simulink model "ryll"  (R2015b)
settings: Solver=FixedStepAuto  StartTime=0  StopTime=8.9  FixedStep=10*(1e-4)  RelTol=1e-3
undefined symbols (not defined in the file or in its folder): qc
libraries: simulink x2
settings Model: Creator=acsl  LastModifiedBy=acsl

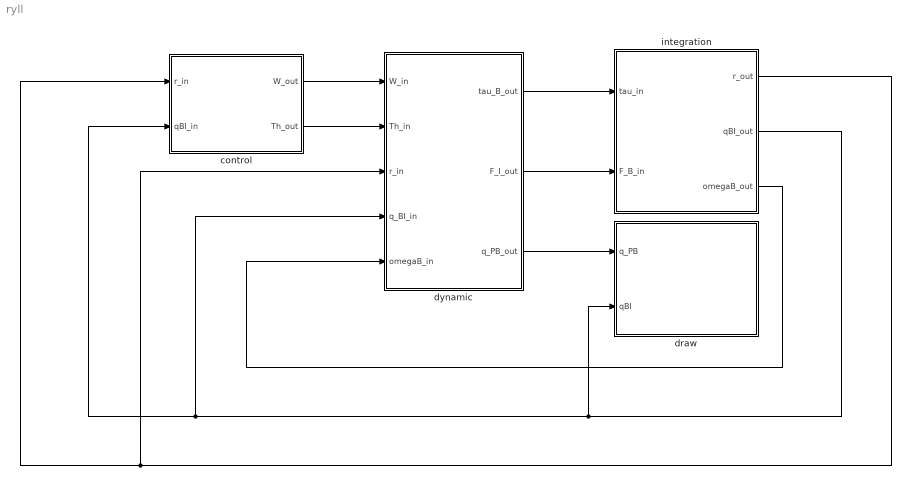
== system ryll ==
  control : Subsystem  InitFcn=init
  draw : Subsystem
  dynamic : Subsystem  StopFcn=close all
  integration : Subsystem
  wires:
  integration/1(r_out) -> dynamic/3(r_in), control/1(r_in)
  control/1(W_out) -> dynamic/1(W_in)
  control/2(Th_out) -> dynamic/2(Th_in)
  dynamic/2(F_I_out) -> integration/2(F_B_in)
  dynamic/1(tau_B_out) -> integration/1(tau_in)
  integration/3(omegaB_out) -> dynamic/5(omegaB_in)
  integration/2(qBI_out) -> draw/2(qBI), dynamic/4(q_BI_in), control/2(qBI_in)
  dynamic/3(q_PB_out) -> draw/1(q_PB)

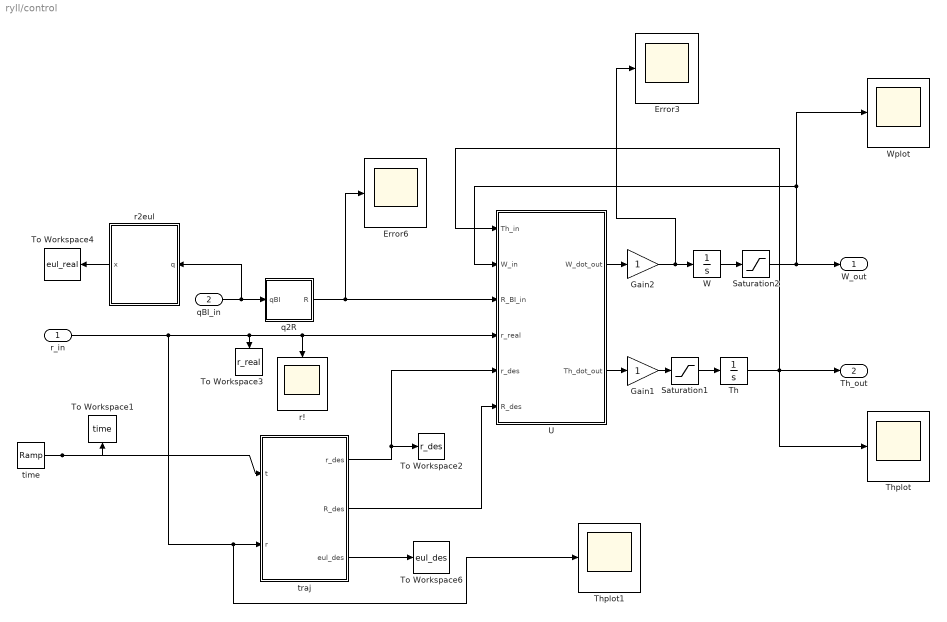
== system ryll/control ==
  r_in : Inport
  qBI_in : Inport  Port=2
  Error3 : Scope
  Error6 : Scope
  Gain1 : Gain
  Gain2 : Gain
  Saturation1 : Saturate  UpperLimit=qc.Th_dot_lim  LowerLimit=-qc.Th_dot_lim
  Saturation2 : Saturate  UpperLimit=qc.W_lim  LowerLimit=-qc.W_lim
  Th : Integrator  InitialCondition=qc.Th0
  Thplot : Scope
  Thplot1 : Scope
  To Workspace1 : ToWorkspace  VariableName=time  SaveFormat=Timeseries  SampleTime=-1
  To Workspace2 : ToWorkspace  VariableName=r_des  SaveFormat=Timeseries  SampleTime=-1
  To Workspace3 : ToWorkspace  VariableName=r_real  SaveFormat=Timeseries  SampleTime=-1
  To Workspace4 : ToWorkspace  VariableName=eul_real  SaveFormat=Timeseries  SampleTime=-1
  To Workspace6 : ToWorkspace  VariableName=eul_des  SaveFormat=Timeseries  SampleTime=-1
  U : Subsystem
  W : Integrator  InitialCondition=qc.W0
  Wplot : Scope
  q2R : MATLAB Function  TreatAsAtomicUnit=on
  r! : Scope
  r2eul : MATLAB Function  TreatAsAtomicUnit=on
  time : simulink/Sources/Ramp  slope=1  start=0  X0=0
  traj : MATLAB Function  TreatAsAtomicUnit=on
  W_out : Outport
  Th_out : Outport  Port=2
  wires:
  U/2(Th_dot_out) -> Gain1/1
  U/1(W_dot_out) -> Gain2/1
  W/1 -> Saturation2/1
  Gain1/1 -> Saturation1/1
  Th/1 -> U/1(Th_in), Th_out/1, Thplot/1
  Saturation1/1 -> Th/1
  Gain2/1 -> Error3/1, W/1
  time/1 -> traj/1(t), To Workspace1/1
  traj/2(R_des) -> U/6(R_des)
  q2R/1(R) -> Error6/1, U/3(R_BI_in)
  r_in/1 -> Thplot1/1, traj/2(r), r!/1, U/4(r_real), To Workspace3/1
  r2eul/1(x) -> To Workspace4/1
  traj/3(eul_des) -> To Workspace6/1
  qBI_in/1 -> r2eul/1(q), q2R/1(qBI)
  traj/1(r_des) -> U/5(r_des), To Workspace2/1
  Saturation2/1 -> U/2(W_in), Wplot/1, W_out/1

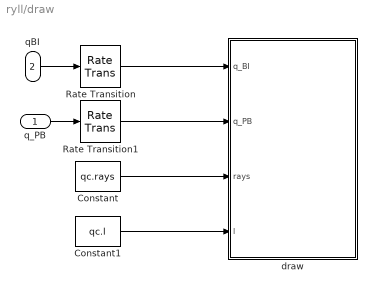
== system ryll/draw ==
  q_PB : Inport
  qBI : Inport  Port=2
  Constant : Constant  Value=qc.rays
  Constant1 : Constant  Value=qc.l
  Rate Transition : RateTransition
  Rate Transition1 : RateTransition
  draw : MATLAB Function  TreatAsAtomicUnit=on  SystemSampleTime=qc.draw_tick
  wires:
  Constant1/1 -> draw/4(l)
  q_PB/1 -> Rate Transition1/1
  Rate Transition1/1 -> draw/2(q_PB)
  Constant/1 -> draw/3(rays)
  Rate Transition/1 -> draw/1(q_BI)
  qBI/1 -> Rate Transition/1

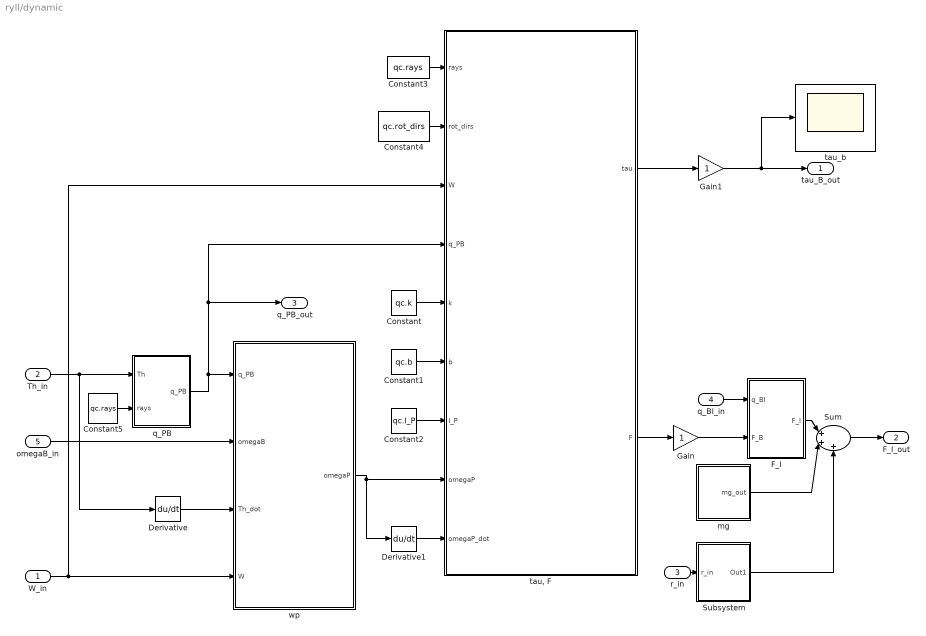
== system ryll/dynamic ==
  W_in : Inport
  Th_in : Inport  Port=2
  r_in : Inport  Port=3
  q_BI_in : Inport  Port=4
  omegaB_in : Inport  Port=5
  Constant : Constant  Value=qc.k
  Constant1 : Constant  Value=qc.b
  Constant2 : Constant  Value=qc.I_P
  Constant3 : Constant  Value=qc.rays
  Constant4 : Constant  Value=qc.rot_dirs
  Constant5 : Constant  Value=qc.rays
  Derivative : Derivative
  Derivative1 : Derivative
  F_I : MATLAB Function  TreatAsAtomicUnit=on
  Gain : Gain
  Gain1 : Gain
  Subsystem : Subsystem
  Sum : Sum  Inputs=|+++
  mg : Subsystem
  q_PB : MATLAB Function  TreatAsAtomicUnit=on
  "tau, F" : MATLAB Function  TreatAsAtomicUnit=on
  tau_b : Scope
  wp : MATLAB Function  TreatAsAtomicUnit=on
  tau_B_out : Outport
  F_I_out : Outport  Port=2
  q_PB_out : Outport  Port=3
  wires:
  Th_in/1 -> q_PB/1(Th), Derivative/1
  q_PB/1(q_PB) -> "tau, F"/4(q_PB), q_PB_out/1, wp/1(q_PB)
  omegaB_in/1 -> wp/2(omegaB)
  Derivative/1 -> wp/3(Th_dot)
  W_in/1 -> "tau, F"/3(W), wp/4(W)
  wp/1(omegaP) -> Derivative1/1, "tau, F"/8(omegaP)
  Constant/1 -> "tau, F"/5(k)
  Constant1/1 -> "tau, F"/6(b)
  Constant2/1 -> "tau, F"/7(I_P)
  "tau, F"/2(F) -> Gain/1
  Constant3/1 -> "tau, F"/1(rays)
  Constant4/1 -> "tau, F"/2(rot_dirs)
  Gain1/1 -> tau_b/1, tau_B_out/1
  Constant5/1 -> q_PB/2(rays)
  q_BI_in/1 -> F_I/1(q_BI)
  Gain/1 -> F_I/2(F_B)
  F_I/1(F_I) -> Sum/1
  mg/1(mg_out) -> Sum/2
  Sum/1 -> F_I_out/1
  r_in/1 -> Subsystem/1(r_in)
  Subsystem/1(Out1) -> Sum/3
  "tau, F"/1(tau) -> Gain1/1
  Derivative1/1 -> "tau, F"/9(omegaP_dot)

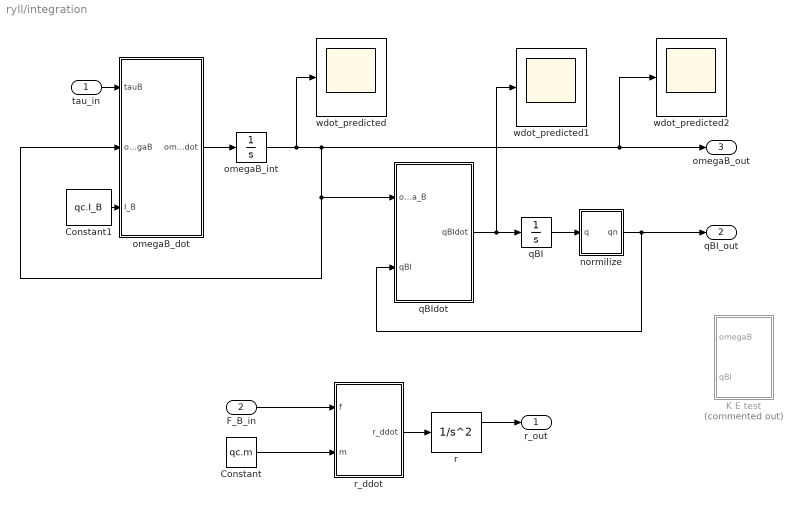
== system ryll/integration ==
  tau_in : Inport
  F_B_in : Inport  Port=2
  Constant : Constant  Value=qc.m
  Constant1 : Constant  Value=qc.I_B
  K E test : Subsystem  Commented=on
  normilize : MATLAB Function  TreatAsAtomicUnit=on
  omegaB_dot : MATLAB Function  TreatAsAtomicUnit=on
  omegaB_int : Integrator  InitialCondition=qc.omegaB0
  qBI : Integrator  InitialCondition=qc.qBI0
  qBIdot : MATLAB Function  TreatAsAtomicUnit=on
  r : SecondOrderIntegrator  ICX=qc.r0
  r_ddot : MATLAB Function  TreatAsAtomicUnit=on
  wdot_predicted : Scope
  wdot_predicted1 : Scope
  wdot_predicted2 : Scope
  r_out : Outport
  qBI_out : Outport  Port=2
  omegaB_out : Outport  Port=3
  wires:
  r/1 -> r_out/1
  r_ddot/1(r_ddot) -> r/1
  Constant/1 -> r_ddot/2(m)
  omegaB_int/1 -> wdot_predicted/1, wdot_predicted2/1, omegaB_out/1, qBIdot/1(omega_B), omegaB_dot/2(omegaB)
  Constant1/1 -> omegaB_dot/3(I_B)
  tau_in/1 -> omegaB_dot/1(tauB)
  qBIdot/1(qBIdot) -> wdot_predicted1/1, qBI/1
  qBI/1 -> normilize/1(q)
  normilize/1(qn) -> qBI_out/1, qBIdot/2(qBI)
  F_B_in/1 -> r_ddot/1(f)
  omegaB_dot/1(omegaB_dot) -> omegaB_int/1

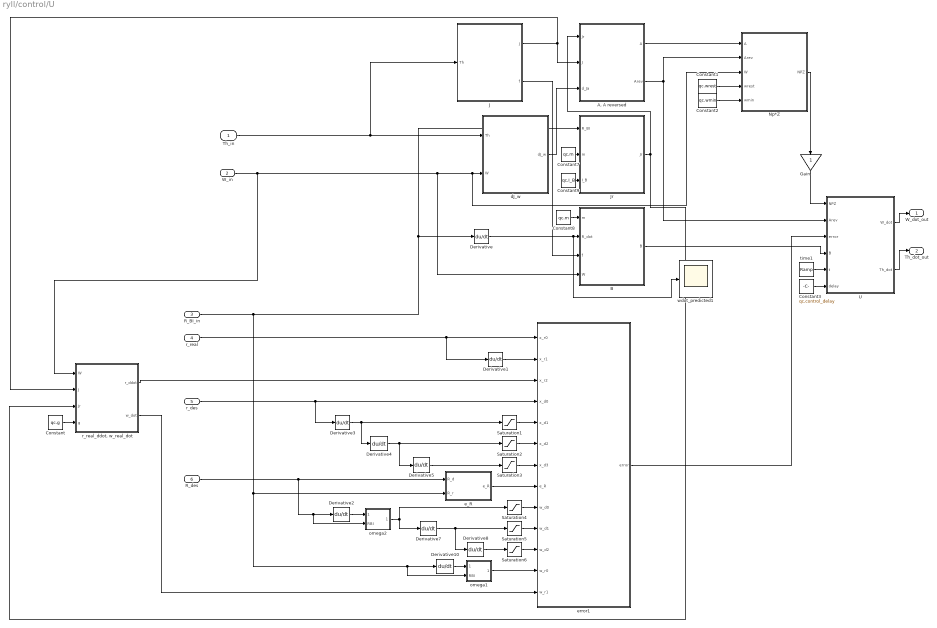
== system ryll/control/U ==
  Th_in : Inport
  W_in : Inport  Port=2
  R_BI_in : Inport  Port=3
  r_real : Inport  Port=4
  r_des : Inport  Port=5
  R_des : Inport  Port=6
  "A, A reversed" : MATLAB Function  TreatAsAtomicUnit=on
  B : MATLAB Function  TreatAsAtomicUnit=on
  Constant : Constant  Value=qc.g
  Constant1 : Constant  Value=qc.wrest
  Constant2 : Constant  Value=qc.wmin
  Constant3 : Constant  Value=qc.control_delay
  Constant7 : Constant  Value=qc.m
  Constant8 : Constant  Value=qc.m
  Constant9 : Constant  Value=qc.I_B
  Derivative{,1..5,7..8,10} (9 alike) : Derivative
  Gain : Gain
  J : MATLAB Function  TreatAsAtomicUnit=on
  Jr : MATLAB Function  TreatAsAtomicUnit=on
  Np*Z : MATLAB Function  TreatAsAtomicUnit=on
  Saturation1 : Saturate  UpperLimit=qc.r_sat_lim  LowerLimit=-qc.r_sat_lim
  Saturation2 : Saturate  UpperLimit=qc.r_sat_lim  LowerLimit=-qc.r_sat_lim
  Saturation3 : Saturate  UpperLimit=qc.r_sat_lim  LowerLimit=-qc.r_sat_lim
  Saturation4 : Saturate  UpperLimit=qc.w_des_sat_lim  LowerLimit=-qc.w_des_sat_lim
  Saturation5 : Saturate  UpperLimit=qc.w_des_sat_lim  LowerLimit=-qc.w_des_sat_lim
  Saturation6 : Saturate  UpperLimit=qc.w_des_sat_lim  LowerLimit=-qc.w_des_sat_lim
  U : MATLAB Function  TreatAsAtomicUnit=on
  dJ_w : MATLAB Function  TreatAsAtomicUnit=on
  e_R : MATLAB Function  TreatAsAtomicUnit=on
  error1 : MATLAB Function  TreatAsAtomicUnit=on
  omega1 : MATLAB Function  TreatAsAtomicUnit=on
  omega2 : MATLAB Function  TreatAsAtomicUnit=on
  "r_real_ddot, w_real_dot" : MATLAB Function  TreatAsAtomicUnit=on
  time1 : simulink/Sources/Ramp  slope=1  start=0  X0=0
  wdot_predicted1 : Scope
  W_dot_out : Outport
  Th_dot_out : Outport  Port=2
  wires:
  Constant9/1 -> Jr/3(I_B)
  Constant8/1 -> B/1(m)
  Constant7/1 -> Jr/2(m)
  Th_in/1 -> J/1(Th), dJ_w/1(Th)
  W_in/1 -> Np*Z/3(W), dJ_w/2(W), B/4(W), "r_real_ddot, w_real_dot"/1(W)
  dJ_w/1(dJ_w) -> "A, A reversed"/3(d_Ja)
  Jr/1(Jr) -> "r_real_ddot, w_real_dot"/3(Jr), "A, A reversed"/1(Jr)
  J/2(f) -> B/3(f)
  J/1(J) -> "A, A reversed"/2(J), "r_real_ddot, w_real_dot"/2(J)
  "A, A reversed"/2(Arev) -> U/2(Arev), Np*Z/2(Arev)
  B/1(B) -> U/4(B)
  U/1(W_dot) -> W_dot_out/1
  U/2(Th_dot) -> Th_dot_out/1
  "A, A reversed"/1(A) -> Np*Z/1(A)
  Constant1/1 -> Np*Z/4(wrest)
  Constant2/1 -> Np*Z/5(wmin)
  r_real/1 -> error1/1(x_r0), Derivative1/1
  Derivative1/1 -> error1/2(x_r1)
  R_des/1 -> omega2/2(RBI), Derivative2/1, e_R/1(R_d)
  e_R/1(e_R) -> error1/8(e_R)
  Derivative10/1 -> omega1/1(RBIdot)
  Derivative3/1 -> Saturation1/1, Derivative4/1
  Constant/1 -> "r_real_ddot, w_real_dot"/4(g)
  error1/1(error) -> U/3(error)
  Np*Z/1(NPZ) -> Gain/1
  R_BI_in/1 -> e_R/2(R_r), omega1/2(RBI), Derivative10/1, Derivative/1, Jr/1(R_BI)
  omega1/1(omega) -> error1/12(w_r0)
  Derivative2/1 -> omega2/1(RBIdot)
  Derivative4/1 -> Saturation2/1, Derivative5/1
  Derivative5/1 -> Saturation3/1
  "r_real_ddot, w_real_dot"/1(r_ddot) -> error1/3(x_r2)
  omega2/1(omega) -> Saturation4/1, Derivative7/1
  Derivative7/1 -> Saturation5/1, Derivative8/1
  Derivative8/1 -> Saturation6/1
  "r_real_ddot, w_real_dot"/2(w_dot) -> error1/13(w_r1)
  Derivative/1 -> wdot_predicted1/1, B/2(R_dot)
  time1/1 -> U/5(t)
  Gain/1 -> U/1(NPZ)
  r_des/1 -> error1/4(x_d0), Derivative3/1
  Saturation1/1 -> error1/5(x_d1)
  Saturation2/1 -> error1/6(x_d2)
  Saturation3/1 -> error1/7(x_d3)
  Constant3/1 -> U/6(delay)
  Saturation4/1 -> error1/9(w_d0)
  Saturation5/1 -> error1/10(w_d1)
  Saturation6/1 -> error1/11(w_d2)

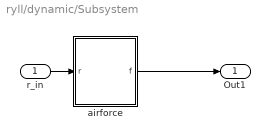
== system ryll/dynamic/Subsystem ==
  r_in : Inport
  airforce : Subsystem
  Out1 : Outport
  wires:
  r_in/1 -> airforce/1(r)
  airforce/1(f) -> Out1/1

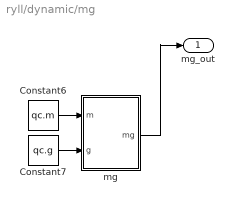
== system ryll/dynamic/mg ==
  Constant6 : Constant  Value=qc.m
  Constant7 : Constant  Value=qc.g
  mg : MATLAB Function  TreatAsAtomicUnit=on
  mg_out : Outport
  wires:
  Constant7/1 -> mg/2(g)
  Constant6/1 -> mg/1(m)
  mg/1(mg) -> mg_out/1

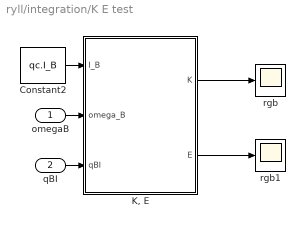
== system ryll/integration/K E test ==
  omegaB : Inport
  qBI : Inport  Port=2
  Constant2 : Constant  Value=qc.I_B
  "K, E" : MATLAB Function  TreatAsAtomicUnit=on
  rgb : Scope
  rgb1 : Scope
  wires:
  omegaB/1 -> "K, E"/2(omega_B)
  qBI/1 -> "K, E"/3(qBI)
  "K, E"/1(K) -> rgb/1
  "K, E"/2(E) -> rgb1/1
  Constant2/1 -> "K, E"/1(I_B)

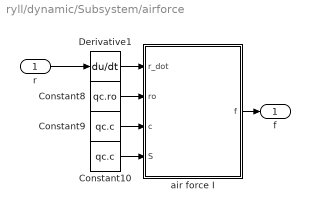
== system ryll/dynamic/Subsystem/airforce ==
  r : Inport
  Constant10 : Constant  Value=qc.c
  Constant8 : Constant  Value=qc.ro
  Constant9 : Constant  Value=qc.c
  Derivative1 : Derivative
  air force I : MATLAB Function  TreatAsAtomicUnit=on
  f : Outport
  wires:
  r/1 -> Derivative1/1
  air force I/1(f) -> f/1
  Constant9/1 -> air force I/3(c)
  Constant10/1 -> air force I/4(S)
  Constant8/1 -> air force I/2(ro)
  Derivative1/1 -> air force I/1(r_dot)

== matlab function ryll/dynamic/wp ==
  data: q_PB input; omegaP output; omegaB input; Th_dot input; W input
function omegaP = fcn(q_PB, omegaB, Th_dot, W)

omegaP = zeros(4*3,1);
for i = 1:4
    q_pb = q_PB(:, i);
    q_bp = quatDual(q_pb);
    w = sign(W(i))*sqrt(abs(W(i)));
    omegaP(3*i-2:3*i, 1) = quatRotate(q_bp, omegaB) + [Th_dot(i); 0; w];
end

== matlab function ryll/integration/normilize ==
  data: q input; qn output
function qn  = fcn(q)
qn = q / norm(q);

== matlab function ryll/dynamic/tau, F ==
  data: rays input; rot_dirs input; W input; q_PB input; k input; b input; I_P input; omegaP input; omegaP_dot input; tau output; F output
function [tau, F]= fcn(rays, rot_dirs, W, q_PB, k, b, I_P, omegaP, omegaP_dot)

tau = [0;0;0];
F = [0;0;0];
Jt2 = zeros(3, 4);
for i = 1:4
    ray = rays(3*i-2:3*i);
    dir = rot_dirs(i);
    omega_p = omegaP(3*i-2:3*i);
    omega_pz = omega_p(3);
    omega_p_dot = omegaP_dot(3*i-2:3*i);
    q_pb = q_PB(:, i);

    fp = dir*[0;0;k*W(i)];
    fb = quatRotate(q_pb,fp);
    
    tau_p_ext = [0;0;-b*abs(omega_pz)*omega_pz];
    tau_p = 1*I_P*omega_p_dot + 1*cross(omega_p, I_P*omega_p) - tau_p_ext;
    tau_b = cross(ray, fb) - quatRotate(q_pb, tau_p);
    
    tau = tau + tau_b;
    
    Jt2(:,i) = tau_b/W(i);
    
    F = F + fb;
end

== matlab function ryll/control/U/J ==
  data: Th input; J output; f output
function [J, f] = fnc(Th)
J = J_fcn(Th(1), Th(2), Th(3), Th(4));
f = J(1:3, 1:4);
end

== matlab function ryll/dynamic/mg/mg ==
  data: m input; mg output; g input
function mg  = fcn(m, g)
mg = m*g;

== matlab function ryll/integration/r_ddot ==
  data: r_ddot output; f input; m input
function r_ddot  = fcn(f, m)

r_ddot = f/m;

== matlab function ryll/control/r2eul ==
  data: q input; x output
function x = fnc(q)
eul = quat2eul(q');
x = eul';
end

== matlab function ryll/integration/omegaB_dot ==
  data: tauB input; omegaB_dot output; omegaB input; I_B input
function omegaB_dot  = fcn(tauB, omegaB, I_B)
omegaB_dot = I_B^(-1) * (tauB - 1*cross(omegaB, I_B * omegaB));

== matlab function ryll/dynamic/F_I ==
  data: q_BI input; F_I output; F_B input
function F_I  = fcn(q_BI, F_B)
F_I = quatRotate(q_BI, F_B);

== matlab function ryll/integration/qBIdot ==
  data: omega_B input; qBIdot output; qBI input
function qBIdot  = fcn(omega_B, qBI)
qw = [0;omega_B];
qBIdot = 0.5*quatMultiply(qBI, qw);

== matlab function ryll/control/q2R ==
  data: qBI input; R output
function R = q2R(qBI)
R = quat2matrix(qBI);
end

== matlab function ryll/draw/draw ==
  data: q_BI input; q_PB input; rays input; l input
function fcn(q_BI, q_PB, rays, l)
hold on
cla(gca)
%% rays and propellers axis
m = 0.25;
for i = 1:4
    ray = rays(3*i-2:3*i);
    ray_rotated = quatRotate(q_BI, ray);
    line ([0 ray_rotated(1)], [0 ray_rotated(2)], [0 ray_rotated(3)], 'color', 'k', 'linestyle', '-')
    
    % propeller axis
    ex = [1;0;0]*l*m;
    ey = [0;1;0]*l*m;
    ez = [0;0;1]*l*m;
    q_pb = q_PB(:, i);
    x =  quatRotate(q_BI, quatRotate(q_pb, ex));
    y =  quatRotate(q_BI, quatRotate(q_pb, ey));
    z =  quatRotate(q_BI, quatRotate(q_pb, ez));
    line ([ray_rotated(1) x(1)+ray_rotated(1)], [ray_rotated(2) x(2)+ray_rotated(2)], [ray_rotated(3) x(3)+ray_rotated(3)], 'color', 'r')
    line ([ray_rotated(1) y(1)+ray_rotated(1)], [ray_rotated(2) y(2)+ray_rotated(2)], [ray_rotated(3) y(3)+ray_rotated(3)], 'color', 'g')
    line ([ray_rotated(1) z(1)+ray_rotated(1)], [ray_rotated(2) z(2)+ray_rotated(2)], [ray_rotated(3) z(3)+ray_rotated(3)], 'color', 'b')
end

%% circle
step = 0.1;
ang=0:step:2*pi + step; 
xp=l*cos(ang);
yp=l*sin(ang);
s = size(xp);
xp_rotated = zeros(1, s(2));
yp_rotated = zeros(1, s(2));
zp_rotated = zeros(1, s(2));
for i = 1:s(2)
    rp = [xp(i);yp(i);0];   
    rp_rotated = quatRotate(q_BI, rp);
    xp_rotated(1, i) = rp_rotated(1);
    yp_rotated(1, i) = rp_rotated(2);
    zp_rotated(1, i) = rp_rotated(3);
end
plot3(xp_rotated,yp_rotated,zp_rotated);

%% body axis
m = 1/2;
ex = [1;0;0]*l*m;
ey = [0;1;0]*l*m;
ez = [0;0;1]*l*m;

x = quatRotate(q_BI, ex);
y = quatRotate(q_BI, ey);
z = quatRotate(q_BI, ez);

line ([0 x(1)], [0 x(2)], [0 x(3)], 'color', 'r')
line ([0 y(1)], [0 y(2)], [0 y(3)], 'color', 'g')
line ([0 z(1)], [0 z(2)], [0 z(3)], 'color', 'b')

%% draw
scale = l*1.5;
axis([-scale scale -scale scale -scale scale]);
xlabel('x');
ylabel('y');
zlabel('z');

== matlab function ryll/integration/K E test/K, E ==
  data: I_B input; omega_B input; qBI input; K output; E output
function [K, E] = fcn(I_B, omega_B, qBI)
K_B = I_B*omega_B;
K = quatRotate(qBI, K_B);
E = omega_B'*I_B*omega_B / 2;

== matlab function ryll/control/U/dJ_w ==
  data: Th input; W input; dJ_w output
function dJ_w = fcn(Th, W)
    dJ_w = dJ_w_fcn(Th(1), Th(2), Th(3), Th(4), W(1), W(2), W(3), W(4));
end

== matlab function ryll/control/U/Jr ==
  data: R_BI input; Jr output; m input; I_B input

function Jr = fcn(R_BI, m, I_B)
Jr = [(1/m)*R_BI zeros(3);
      zeros(3) I_B^(-1)];
end

== matlab function ryll/control/U/A, A reversed ==
  data: Jr input; J input; d_Ja input; A output; Arev output
function [A, Arev] = fcn(Jr, J, d_Ja)
A = Jr * [J d_Ja];
Arev = pinv(A);
end

== matlab function ryll/control/U/B ==
  data: m input; R_dot input; f input; B output; W input
function B  = fcn(m, R_dot, f, W)
B = [(1/m)*R_dot*f*W; zeros(3,1)];
end

== matlab function ryll/control/U/Np*Z ==
  data: A input; Arev input; NPZ output; W input; wrest input; wmin input
function NPZ  = fcn(A, Arev, W, wrest, wmin)
kh1 = 1*1e2;
kh2 = 1*1e-2;
k = 1;

Z = zeros(8,1);
for i=1:4
    w = abs(W(i));
    if w > wrest
        Z(i) = kh2*(2*w - 2*wrest);
    elseif w > wmin
        Z(i) = (2*kh1*pi*tan((w*pi)/(2*wmin - 2*wrest) - (wrest*pi)/(2*wmin - 2*wrest))*(tan((w*pi)/(2*wmin - 2*wrest) - (wrest*pi)/(2*wmin - 2*wrest))^2 + 1))/(2*wmin - 2*wrest);
    else
        Z(i) = 0;
    end
    Z(i) = -Z(i)*sign(W(i));
end
NPZ = (eye(8) - Arev*A) * Z;
end

== matlab function ryll/control/U/omega2 ==
  data: omega output; RBIdot input; RBI input
function omega  = fcn(RBIdot, RBI)

R = RBI'*RBIdot;
omega = [-R(2,3); R(1,3); -R(1,2)];

== matlab function ryll/control/U/U ==
  data: NPZ input; Arev input; error input; B input; W_dot output; Th_dot output; t input; delay input
function [W_dot, Th_dot]   = fcn(NPZ, Arev, error, B, t, delay)
U = zeros(8, 1);
if t > delay
    U = Arev*(error - B) + NPZ;
end
W_dot = U(1:4);
Th_dot = U(5:8);
end

== matlab function ryll/control/U/error1 ==
  data: x_r0 input; x_r1 input; error output; x_r2 input; x_d0 input; x_d1 input; x_d2 input; x_d3 input; e_R input; w_d0 input; w_d1 input; w_d2 input; w_r0 input; w_r1 input
function error = x_e(x_r0, x_r1, x_r2, x_d0, x_d1, x_d2, x_d3, e_R, w_d0, w_d1, w_d2, w_r0, w_r1)
   
K2 = [1,0,0;
      0,1,0;
      0,0,1]*28.5;

K1 = [1,0,0;
      0,1,0;
      0,0,1]*271;

K0 =  [1,0,0;
       0,1,0;
       0,0,1]*857;
   
e_x = 1*x_d3 + K2*(x_d2 - x_r2) + K1*(x_d1 - x_r1)+ K0*(x_d0 - x_r0);
e_x = e_x;

C2 =   [1,0,0;
        0,1,0;
        0,0,1]*45;

C1 =   [1,0,0;
        0,1,0;
        0,0,1]*675;

C0 =   [1,0,0;
        0,1,0;
        0,0,1.6]*3375;
    
% C2 =   [1,0,0;
%     0,1,0;
%     0,0,1]*300;
% 
% C1 =   [1,0,0;
%     0,1,0;
%     0,0,1]*1500;
% 
% C0 =   [1,0,0;
%     0,1,0;
%     0,0,1.6]*6000;
       
e_r = w_d2 + C2*(w_d1 - w_r1) + C1*(w_d0 - w_r0) + C0*(e_R);
e_r = 1*e_r*1;

x = [w_d2,C2*(w_d1 - w_r1),C1*(w_d0 - w_r0),C0*(e_R)];
x = [1*x_d3, K2*(x_d2 - x_r2), K1*(x_d1 - x_r1), K0*(x_d0 - x_r0)];

error = [e_x; e_r];
end

== matlab function ryll/control/U/e_R ==
  data: R_d input; R_r input; e_R output size=3
function e_R = e_r(R_d, R_r)
Me_R = R_r'*R_d - R_d'*R_r;
e_R = 0.5*[-Me_R(2,3); Me_R(1,3); -Me_R(1,2)];
end

== matlab function ryll/control/U/omega1 ==
  data: omega output; RBIdot input; RBI input
function omega  = fcn(RBIdot, RBI)

R = RBI'*RBIdot;
omega = [-R(2,3); R(1,3); -R(1,2)];

== matlab function ryll/control/traj ==
  data: r_des output; R_des output; t input; eul_des output; r input
function [r_des, R_des, eul_des] = curve(t, r)

%% toPoint
% r_des = 20*[1.1;0.7;1.2];
% eul_des = 0*[14;12;8]*pi/180;
% R_des = eul2rotm(eul_des');

% %% camera
% radius = 4;
% period = 2*pi/8;
% phase = 0;
% r_des = 1*[radius*sin(t*period+phase);radius*cos(t*period+phase);0];
% eul_des = 1*[period*t;0*t;0*t];
% R_des = eul2rotm(eul_des');

%% line acc
r_des = [1*t^2;0;0];
q = [1;0;0;0];
R_des = quat2rotm(q');
eul_des = quat2eul(q')';

% %% trees
% 
% v = 3;
% radius = 1.5;
% period = 2*pi*radius/v;
% r_des = [0;0;0];
% dr = [1;0;0];
% if t < 0.5*period
%     phase = -pi;
%     arg = t*2*pi/period + phase;
%     r0 = [0; 0; 0];
%     x = radius*cos(arg) + r0(1);
%     y = radius*sin(arg) + r0(2);
%     r_des = [x;y;0];
%     dr = [-radius*sin(arg); radius*cos(arg); 0];
% elseif t < period
%     phase = 0;
%     arg = -t*2*pi/period + phase;
%     r0 = [2*radius; 0; 0];
%     x = radius*cos(arg) + r0(1);
%     y = radius*sin(arg) + r0(2);
%     r_des = [x;y;0];
%     dr = [radius*sin(arg); -radius*cos(arg); 0];
% elseif t < 2*period
%     phase = -pi;
%     arg = t*2*pi/period + phase;
%     r0 = [4*radius; 0; 0];
%     x = radius*cos(arg) + r0(1);
%     y = radius*sin(arg) + r0(2);
%     r_des = [x;y;0];
%     dr = [-radius*sin(arg); radius*cos(arg); 0];
% elseif t < 2.5*period
%     phase = 0;
%     arg = -t*2*pi/period + phase;
%     r0 = [2*radius; 0; 0];
%     x = radius*cos(arg) + r0(1);
%     y = radius*sin(arg) + r0(2);
%     r_des = [x;y;0];
%     dr = [radius*sin(arg); -radius*cos(arg); 0];
% elseif t < 3*period
%     phase = -pi;
%     arg = t*2*pi/period + phase;
%     r0 = [0; 0; 0];
%     x = radius*cos(arg) + r0(1);
%     y = radius*sin(arg) + r0(2);
%     r_des = [x;y;0];
%     dr = [-radius*sin(arg); radius*cos(arg); 0];
% end
% 
% q = quatBetweenVectors([1;0;0], dr);
% % q = [1;0;0;0];
% R_des = quat2rotm(q');
% eul_des = quat2eul(q')';
end

== matlab function ryll/dynamic/q_PB ==
  data: Th input; q_PB output; rays input
function q_PB = fcn(Th, rays)
ex = [1;0;0];
ez = [0;0;1];
q_PB = zeros(4, 4);
for i = 1:4
    ray = rays(3*i-2:3*i);
    cosAlpha = dot(ex, ray/norm(ray));
    alpha = acos(cosAlpha);
    if(ray(2) < 0)
        alpha = -alpha;
    end
    th = Th(i);
    qth = [cos(th/2);ex*sin(th/2)];
    qa = [cos(alpha/2);ez*sin(alpha/2)];
    q = quatMultiply(qa, qth);
    q_PB(:,i) = q;
end

== matlab function ryll/dynamic/Subsystem/airforce/air force I ==
  data: r_dot input; f output; ro input; c input; S input
function f = fcn(r_dot, ro, c, S)
f = -ro*c*S*norm(r_dot)*r_dot;

== matlab function ryll/control/U/r_real_ddot, w_real_dot ==
  data: W input; J input; Jr input; g input; r_ddot output; w_dot output
function [r_ddot, w_dot]  = fcn(W, J, Jr, g)
f = [g;zeros(3,1)];
s_ddot = f + Jr*J*W;
r_ddot = s_ddot(1:3);
w_dot = s_ddot(4:6);
end
